simulink model "qamwnymf"  (Simulink 7.4)
settings: Solver=ode45  StartTime=0.0  StopTime=999999  MaxStep=0.05  MinStep=0.0001  RelTol=1e-6  AbsTol=1e-6
values from neighbouring files (symbols this model uses):
  den = real(poly(p(v:v+1)))    [bwthui.m]    (also in rcosfltk.m = 3)
  num = real(poly(z(index)))    [bwthui.m]    (also in rcosfltk.m = 0.5)
undefined symbols (not defined in the file or in its folder): eyediasi, eyesampl, sbiterr
libraries: librnew x1
(part 2 of 2)

== system qamwnymf/Receiver/Root-RC receive filter_/Memory Impulse/discrete Rising edge detector ==
  in_1 : Inport  OutDataType=sfix(16)  OutScaling=2^0
  Relational Operator : RelationalOperator  InputSameDT=on
  Relational Operator1 : RelationalOperator  InputSameDT=on
  Relational Operator2 : RelationalOperator  Operator=>  InputSameDT=on
  Unit Delay : UnitDelay  SampleTime=ts
  one1 : Constant  Value=thld  OutDataType=sfix(16)  OutScaling=2^0
  out_1 : Outport
  wires:
  Relational Operator2/1 -> out_1/1
  Relational Operator1/1 -> Relational Operator2/2
  Relational Operator/1 -> Relational Operator2/1
  one1/1 -> Relational Operator1/2, Relational Operator/2
  Unit Delay/1 -> Relational Operator1/1
  in_1/1 -> Unit Delay/1, Relational Operator/1

== system qamwnymf/Transmitter/Root-RC transmit filter/Memory Impulse/discrete Rising edge detector ==
  in_1 : Inport  OutDataType=sfix(16)  OutScaling=2^0
  Relational Operator : RelationalOperator  InputSameDT=on
  Relational Operator1 : RelationalOperator  InputSameDT=on
  Relational Operator2 : RelationalOperator  Operator=>  InputSameDT=on
  Unit Delay : UnitDelay  SampleTime=ts
  one1 : Constant  Value=thld  OutDataType=sfix(16)  OutScaling=2^0
  out_1 : Outport
  wires:
  in_1/1 -> Unit Delay/1, Relational Operator/1
  Unit Delay/1 -> Relational Operator1/1
  one1/1 -> Relational Operator1/2, Relational Operator/2
  Relational Operator/1 -> Relational Operator2/1
  Relational Operator1/1 -> Relational Operator2/2
  Relational Operator2/1 -> out_1/1

== system qamwnymf/Transmitter/Root-RC transmit filter_/Memory Impulse/discrete Rising edge detector ==
  in_1 : Inport  OutDataType=sfix(16)  OutScaling=2^0
  Relational Operator : RelationalOperator  InputSameDT=on
  Relational Operator1 : RelationalOperator  InputSameDT=on
  Relational Operator2 : RelationalOperator  Operator=>  InputSameDT=on
  Unit Delay : UnitDelay  SampleTime=ts
  one1 : Constant  Value=thld  OutDataType=sfix(16)  OutScaling=2^0
  out_1 : Outport
  wires:
  in_1/1 -> Unit Delay/1, Relational Operator/1
  Unit Delay/1 -> Relational Operator1/1
  one1/1 -> Relational Operator1/2, Relational Operator/2
  Relational Operator/1 -> Relational Operator2/1
  Relational Operator1/1 -> Relational Operator2/2
  Relational Operator2/1 -> out_1/1
